simulink model "Resonant_Power_Transfer"  (R2025b)
settings: Solver=ode23t  StartTime=0.0  StopTime=2  RelTol=1e-3
undefined symbols (not defined in the file or in its folder): Ion, Lithium
libraries: spsCurrentMeasurementLib x6, spsSeriesRLCBranchLib x6, spsVoltageMeasurementLib x6, spsDiodeLib x4, spsIGBTDiodeLib x4, spsACVoltageSourceLib x1, spsBatteryLib x1, spsMutualInductanceLib x1, spsPWMGeneratorDCDCLib x1, spsUniversalBridgeLib x1, sps_lib x1
settings Model: Creator=User  LastModifiedBy=Rishi

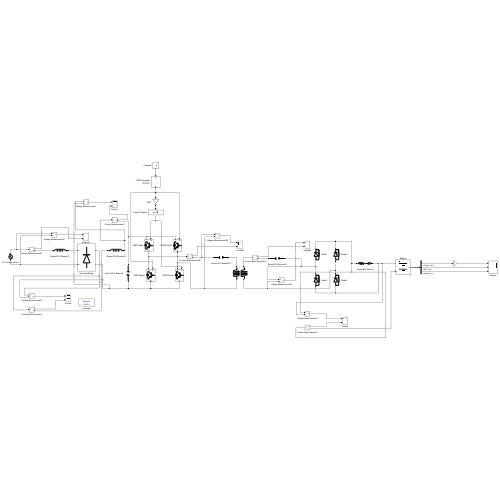
[thumbnail: Simulink's stored preview of the top-level diagram]
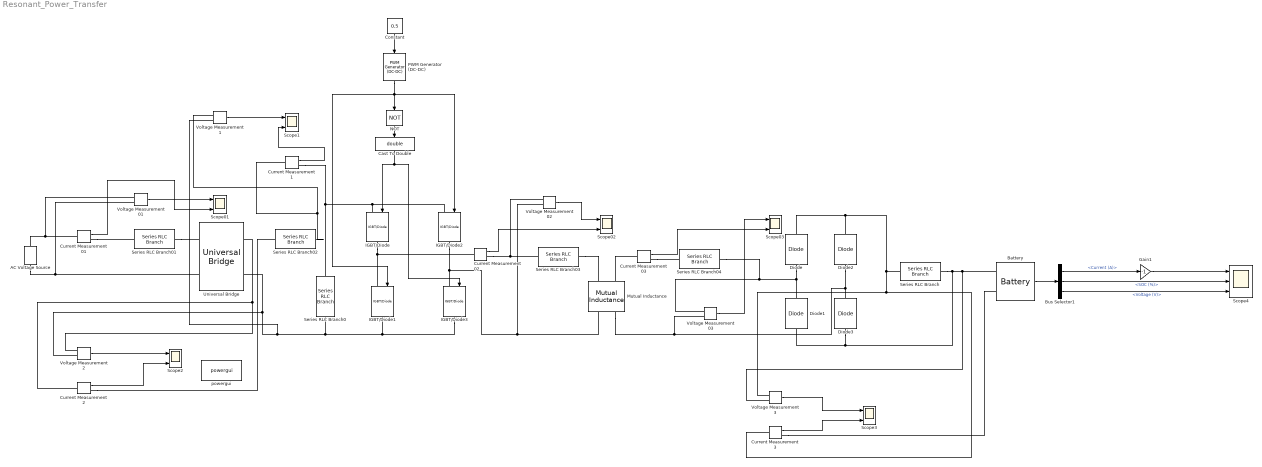
== system Resonant_Power_Transfer ==
  AC Voltage Source : spsACVoltageSourceLib/AC Voltage Source  Amplitude=500  Phase=180  Frequency=60  SampleTime=0  Measurements=Voltage  BusType=swing  Pref=10e3  Qref=0  Qmin=-inf  Qmax=+inf
  Battery : spsBatteryLib/Battery  BatType=Lithium-Ion  NomV=300  NomQ=25  SOC=50  Batt_Tr=2  PresetModel=on  MaxQ=25  MinV=225  FullV=349.1961  Dis_rate=10.8696  R=0.12  Normal_OP=22.6087  expZone="[324.1158      1.228261]"
  Bus Selector1 : BusSelector  OutputSignals=Current (A),SOC (%),Voltage (V)
  Cast To Double : DataTypeConversion  OutDataTypeStr=double  SaturateOnIntegerOverflow=off  RndMeth=Floor
  Constant : Constant  Value=0.5
  Current Measurement01 : spsCurrentMeasurementLib/Current Measurement  PhasorSimulation=off  OutputType=Complex  PSBequivalent=0
  Current Measurement02 : spsCurrentMeasurementLib/Current Measurement  PhasorSimulation=off  OutputType=Complex  PSBequivalent=0
  Current Measurement03 : spsCurrentMeasurementLib/Current Measurement  PhasorSimulation=off  OutputType=Complex  PSBequivalent=0
  Current Measurement1 : spsCurrentMeasurementLib/Current Measurement  PhasorSimulation=off  OutputType=Complex  PSBequivalent=0
  Current Measurement2 : spsCurrentMeasurementLib/Current Measurement  PhasorSimulation=off  OutputType=Complex  PSBequivalent=0
  Current Measurement3 : spsCurrentMeasurementLib/Current Measurement  PhasorSimulation=off  OutputType=Complex  PSBequivalent=0
  Diode{,1..3} (4 alike) : spsDiodeLib/Diode  Ron=0.001  Lon=0  Vf=0.8  IC=0  UseSnubber=0  Rs=500  Cs=250e-9  Measurements=off
  Gain1 : Gain  Gain=-1
  IGBT/Diode{,1..3} (4 alike) : spsIGBTDiodeLib/IGBT//Diode  Ron=1e-3  Rs=1e5  Cs=inf  Measurements=off
  Mutual Inductance : spsMutualInductanceLib/Mutual Inductance  LConnTagsString=a|b  RConnTagsString=A|B  TypeOfMutual=Two or three windings with equal mutual terms  NumberOfWindings=3  SelfImpedance1=[1e-3 266.16e-6]  SelfImpedance2=[1e-3 256.79e-6]  ThreeWindings=off  SelfImpedance3=[ 1.1 1.1e-03]  MutualImpedance=[0 85.46e-6]  InductanceMatrix="[1.0 0.9  0.9 ;  0.9 1.0  0.9;  0.9 0.9 1.0 ] * 1e-3"  ResistanceMatrix="[1.0 0.9  0.9 ;  0.9 1.0  0.9;  0.9 0.9 1.0 ]"  Measurements=None
      settings: LibrarySourceBlock=sps_lib/Passives/Mutual Inductance
  NOT : Logic  Operator=NOT  IconShape=distinctive  AllPortsSameDT=off  OutDataTypeStr=boolean
  PWM Generator (DC-DC) : spsPWMGeneratorDCDCLib/PWM Generator (DC-DC)  Fsw=30000  Ts=0
  Scope01 : Scope  NumInputPorts=2
      settings: ActiveDisplayYMinimum=-625  ActiveDisplayYMaximum=625  DataLoggingVariableName=ScopeData6
  Scope02 : Scope  NumInputPorts=2
      settings: ActiveDisplayYMinimum=-1850.7196777485656  ActiveDisplayYMaximum=1850.3135325519904
  Scope03 : Scope  NumInputPorts=2
      settings: ActiveDisplayYMinimum=-815.28914764934677  ActiveDisplayYMaximum=815.28932532060583  DataLoggingVariableName=ScopeData2
  Scope1 : Scope  NumInputPorts=2
      settings: ActiveDisplayYMinimum=-9.0485825710013916  ActiveDisplayYMaximum=81.437243170428459
  Scope2 : Scope  NumInputPorts=2
      settings: ActiveDisplayYMinimum=-7.5468267059062777  ActiveDisplayYMaximum=67.763020101162539  DataLoggingVariableName=ScopeData3
  Scope3 : Scope  NumInputPorts=2
      settings: ActiveDisplayYMinimum=-81.326925096664567  ActiveDisplayYMaximum=731.94232586998123  DataLoggingVariableName=ScopeData5
  Scope4 : Scope  NumInputPorts=3
      settings: ActiveDisplayYMinimum=-4637.5965307449069  ActiveDisplayYMaximum=4142.2635254316565  DataLoggingVariableName=ScopeData7
  Series RLC Branch : spsSeriesRLCBranchLib/Series RLC Branch  LConnTagsString=__new0  RConnTagsString=__new0  BranchType=RC  Resistance=0.1  Inductance=1e-3  SetiL0=off  InitialCurrent=0  Capacitance=300e-6  Setx0=off  InitialVoltage=0  Measurements=None
  Series RLC Branch0 : spsSeriesRLCBranchLib/Series RLC Branch  LConnTagsString=__new0  RConnTagsString=__new0  BranchType=C  Resistance=1  Inductance=1e-3  SetiL0=off  InitialCurrent=0  Capacitance=300e-6  Setx0=off  InitialVoltage=0  Measurements=None
  Series RLC Branch01 : spsSeriesRLCBranchLib/Series RLC Branch  LConnTagsString=__new0  RConnTagsString=__new0  BranchType=L  Resistance=1  Inductance=100e-3  SetiL0=off  InitialCurrent=0  Capacitance=1e-6  Setx0=off  InitialVoltage=0  Measurements=None
  Series RLC Branch02 : spsSeriesRLCBranchLib/Series RLC Branch  LConnTagsString=__new0  RConnTagsString=__new0  BranchType=L  Resistance=1  Inductance=10e-3  SetiL0=off  InitialCurrent=0  Capacitance=1e-8  Setx0=off  InitialVoltage=0  Measurements=None
  Series RLC Branch03 : spsSeriesRLCBranchLib/Series RLC Branch  LConnTagsString=__new0  RConnTagsString=__new0  BranchType=C  Resistance=1  Inductance=1e-3  SetiL0=off  InitialCurrent=0  Capacitance=105.74e-9  Setx0=off  InitialVoltage=0  Measurements=None
  Series RLC Branch04 : spsSeriesRLCBranchLib/Series RLC Branch  LConnTagsString=__new0  RConnTagsString=__new0  BranchType=C  Resistance=1  Inductance=1e-3  SetiL0=off  InitialCurrent=0  Capacitance=109.69e-9  Setx0=off  InitialVoltage=0  Measurements=None
  Universal Bridge : spsUniversalBridgeLib/Universal Bridge  Arms=2  SnubberResistance=1e5  SnubberCapacitance=inf  Device=Diodes  Ron=1e-3  Lon=0  ForwardVoltages="[  0  0  ]"  ForwardVoltage=0  GTOparameters=[ 10e-6 , 20e-6 ]  IGBTparameters=[ 1e-6 , 2e-6 ]  Measurements=All voltages and currents  Measurements_2=None  converterType=Rectifier
  Voltage Measurement01 : spsVoltageMeasurementLib/Voltage Measurement  PhasorSimulation=off  OutputType=Complex  PSBequivalent=0
  Voltage Measurement02 : spsVoltageMeasurementLib/Voltage Measurement  PhasorSimulation=off  OutputType=Complex  PSBequivalent=0
  Voltage Measurement03 : spsVoltageMeasurementLib/Voltage Measurement  PhasorSimulation=off  OutputType=Complex  PSBequivalent=0
  Voltage Measurement1 : spsVoltageMeasurementLib/Voltage Measurement  PhasorSimulation=off  OutputType=Complex  PSBequivalent=0
  Voltage Measurement2 : spsVoltageMeasurementLib/Voltage Measurement  PhasorSimulation=off  OutputType=Complex  PSBequivalent=0
  Voltage Measurement3 : spsVoltageMeasurementLib/Voltage Measurement  PhasorSimulation=off  OutputType=Complex  PSBequivalent=0
  powergui : sps_lib/powergui  Priority=1  SimulationMode=Discrete  SampleTime=1e-6  frequency=60  Iterations=50  frequencyindice=0  Pbase=100e6  ErrMax=1e-4  UnitsV=kV  UnitsW=MW  buscounter=0  FunctionMessages=off  echomessages=off  EnableUseOfTLC=off  CurrentSourceSwitches=off  DisableSnubberDevices=off  DisableRonSwitches=off  DisableVfSwitches=off  DisplayEquations=off  AutomaticDiscreteSolvers=off  SolverType=Tustin/Backward Euler (TBE)  Interpol=off  ExternalGateDelay=off  methode=off  Ts=100  x0status=blocks  SPID=on  SwTol=0  HookPort=off  NonlinearTolerance=1e-4  nMaxIteration=100  ContinueOnMaxIteration=off  RestoreLinks=warning  ResistiveCurrentMeasurement=off  Frange=[0:2:500]  Ylog=off  Xlog=on  ShowGrid=off  save=off  variable=ZData  structure=0  ZoomFFT=off  StartTime=0.0  cycles=1  DisplayStyle=1  fundamental=60  FreqAxis=off  MaxFrequency=1000  frequencyindicesteady=1  RmsSteady=1  display=off
  wires:
  Current Measurement02/1 -> Scope02/2
  Current Measurement03/1 -> Scope03/2
  Voltage Measurement03/1 -> Scope03/1
  Constant/1 -> PWM Generator (DC-DC)/1
  PWM Generator (DC-DC)/1 -> IGBT/Diode1/1, IGBT/Diode2/1, NOT/1
  NOT/1 -> Cast To Double/1
  Current Measurement01/1 -> Scope01/2
  Voltage Measurement01/1 -> Scope01/1
  Voltage Measurement02/1 -> Scope02/1
  Cast To Double/1 -> IGBT/Diode/1, IGBT/Diode3/1
  Current Measurement1/1 -> Scope1/2
  Voltage Measurement1/1 -> Scope1/1
  Voltage Measurement2/1 -> Scope2/1
  Current Measurement2/1 -> Scope2/2
  Voltage Measurement3/1 -> Scope3/1
  Current Measurement3/1 -> Scope3/2
  Bus Selector1/1 -> Gain1/1  "<Current (A)>"
  Battery/1 -> Bus Selector1/1
  Bus Selector1/2 -> Scope4/2  "<SOC (%)>"
  Bus Selector1/3 -> Scope4/3  "<Voltage (V)>"
  Gain1/1 -> Scope4/1
  connections:
  Voltage Measurement02/LConn2 -- IGBT/Diode2/RConn1 -- IGBT/Diode3/LConn1 -- Mutual Inductance/RConn1
  IGBT/Diode/RConn1 -- Current Measurement02/LConn1 -- IGBT/Diode1/LConn1
  Diode2/LConn1 -- Mutual Inductance/RConn2 -- Voltage Measurement03/LConn2 -- Diode3/RConn1
  Diode/LConn1 -- Voltage Measurement03/LConn1 -- Series RLC Branch04/RConn1 -- Diode1/RConn1
  Diode3/LConn1 -- Series RLC Branch/RConn1 -- Voltage Measurement3/LConn2 -- Battery/LConn2 -- Diode1/LConn1
  Series RLC Branch03/RConn1 -- Mutual Inductance/LConn1
  Current Measurement02/RConn1 -- Series RLC Branch03/LConn1 -- Voltage Measurement02/LConn1
  Current Measurement03/LConn1 -- Mutual Inductance/LConn2
  Current Measurement03/RConn1 -- Series RLC Branch04/LConn1
  IGBT/Diode3/RConn1 -- IGBT/Diode1/RConn1 -- Series RLC Branch0/RConn1 -- Voltage Measurement1/LConn2 -- Universal Bridge/RConn2 -- Voltage Measurement2/LConn2
  IGBT/Diode2/LConn1 -- Series RLC Branch0/LConn1 -- Current Measurement1/RConn1 -- IGBT/Diode/LConn1
  Diode2/RConn1 -- Current Measurement3/LConn1 -- Voltage Measurement3/LConn1 -- Series RLC Branch/LConn1 -- Diode/RConn1
  AC Voltage Source/LConn1 -- Universal Bridge/LConn2 -- Voltage Measurement01/LConn2
  Current Measurement2/LConn1 -- Voltage Measurement2/LConn1 -- Universal Bridge/RConn1
  Series RLC Branch01/RConn1 -- Universal Bridge/LConn1
  Voltage Measurement01/LConn1 -- Current Measurement01/LConn1 -- AC Voltage Source/RConn1
  Series RLC Branch02/RConn1 -- Current Measurement1/LConn1 -- Voltage Measurement1/LConn1
  Current Measurement01/RConn1 -- Series RLC Branch01/LConn1
  Current Measurement3/RConn1 -- Battery/LConn1
  Current Measurement2/RConn1 -- Series RLC Branch02/LConn1
